simulink model "HeadingHoldControl"  (R2018b)
settings: Solver=VariableStepAuto  StartTime=0.0  StopTime=30  RelTol=1e-3
settings Model: Creator=cdjsd  LastModifiedBy=cdjsd

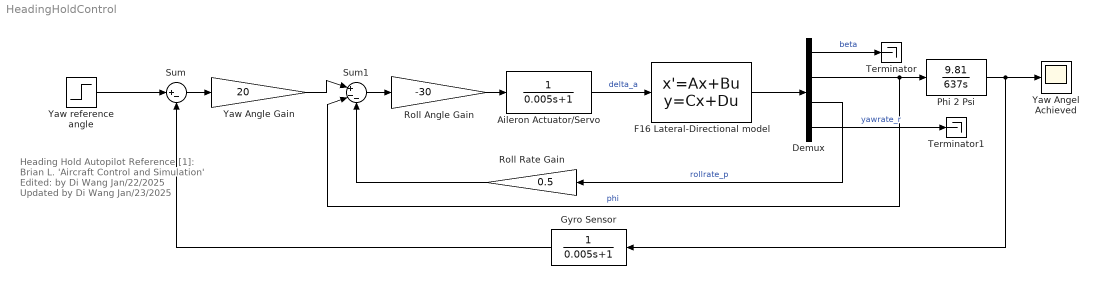
== system HeadingHoldControl ==
  note: Heading Hold Autopilot
      | Reference [1]: Brian L. 'Aircraft Control and Simulation'
      | Edited: by Di Wang Jan/22/2025
      | Updated by Di Wang Jan/23/2025
  Aileron Actuator/Servo : TransferFcn  Denominator=[0.005 1]
  Demux : Demux
  F16 Lateral-Directional model : StateSpace  A=|  B=|  C=eye(4)  D=zeros(4,1)  InitialCondition=0
      A=|
      | [-0.1315 0.14858 0.32434 -0.93964;
      |      0 0 1 0.33976;
      |      -10.614 0 -1.1793 1.0023;
      |      0.99655 0 -0.00182 -0.25855]
      B=|
      | [0.00012;
      |      0;
      |      -0.10316;
      |      -0.00213]
  Gyro Sensor : TransferFcn  Numerator=[0 1]  Denominator=[0.005 1]
  Phi 2 Psi : TransferFcn  Numerator=[9.81]  Denominator=[637 0]
  Roll Angle Gain : Gain  Gain=-30
  Roll Rate Gain : Gain  Gain=0.5
  Sum : Sum  Inputs=|+-
  Sum1 : Sum  Inputs=|+--
  Terminator : Terminator
  Terminator1 : Terminator
  Yaw Angel Achieved : Scope
  Yaw Angle Gain : Gain  Gain=20
  Yaw reference angle : Step  SampleTime=0
  wires:
  Yaw reference angle/1 -> Sum/1
  Sum/1 -> Yaw Angle Gain/1
  F16 Lateral-Directional model/1 -> Demux/1
  Yaw Angle Gain/1 -> Sum1/1
  Sum1/1 -> Roll Angle Gain/1
  Roll Angle Gain/1 -> Aileron Actuator/Servo/1
  Aileron Actuator/Servo/1 -> F16 Lateral-Directional model/1  "delta_a"
  Demux/1 -> Terminator/1  "beta"
  Demux/2 -> Sum1/2, Phi 2 Psi/1  "phi"
  Demux/3 -> Roll Rate Gain/1  "rollrate_p"
  Demux/4 -> Terminator1/1  "yawrate_r"
  Phi 2 Psi/1 -> Gyro Sensor/1, Yaw Angel Achieved/1
  Roll Rate Gain/1 -> Sum1/3
  Gyro Sensor/1 -> Sum/2
